simulink library "OutputBlocks_library"  (R2018b)
settings: Solver=VariableStepAuto  StartTime=0.0  StopTime=10.0  RelTol=1e-3
undefined symbols (not defined in the file): aircraft
libraries: unit_conversions_lib x8, flight_parameters_lib x3, vlm_wing_lib x3, axes_transformation_lib x2, sensors_lib x1, flight_dynamics_models x1
settings Model: ModifiedByFormat=dcava  Creator=cava_da  LastModifiedBy=dcava
settings DataIOCC: ReturnWorkspaceOutputs=on

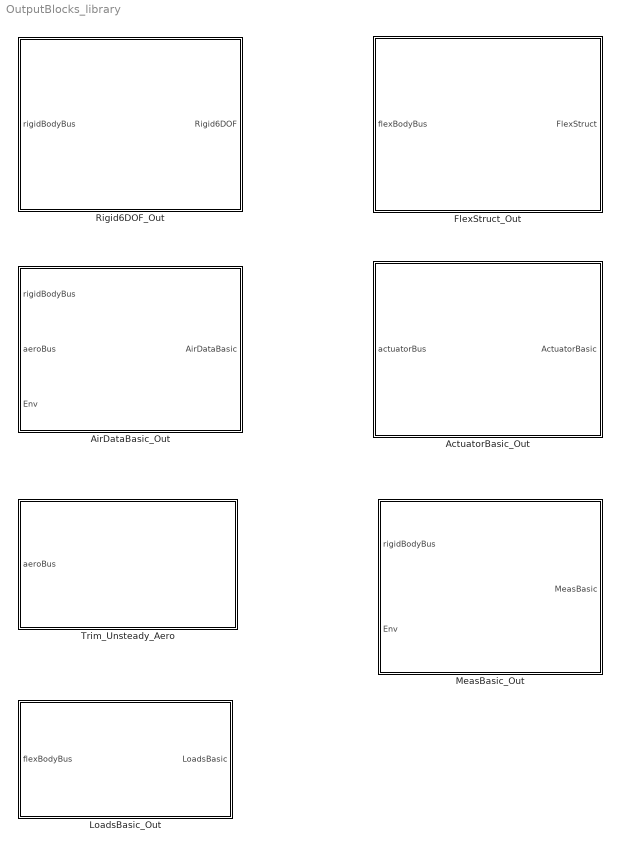
== system OutputBlocks_library ==
  ActuatorBasic_Out : Subsystem  mask{n_ail_pairs=aircraft.wing_main.params.num_flaps/2}
      mask prompts: n_ail_pairs "Number of aileron pairs:"
  AirDataBasic_Out : Subsystem  mask(AirDataBasic_Out){}
      mask DialogControl DescGroupVar Prompt: Air Data Basic
  FlexStruct_Out : Subsystem  mask(FlexStruct_Out){structure_order=size(aircraft.eom_flexible.structure_red.K,2)-6.}
      mask prompts: structure_order "Structural model order"
      mask DialogControl DescGroupVar Prompt: FlexStruct_Out
  LoadsBasic_Out : Subsystem  mask(LoadsBasic_Out){struct_order=size(aircraft.eom_flexible.structure_red.K,2)-6., phi_loads=aircraft.outputs.loads.phi}
      mask prompts: struct_order "Structural model order"; phi_loads "Load transformation matrix (phi)"
  MeasBasic_Out : Subsystem  mask(Rigid6DOF_Out){}
  Rigid6DOF_Out : Subsystem  mask(Rigid6DOF_Out){}
  Trim_Unsteady_Aero : Subsystem  mask{aircraft=aircraft}
      mask prompts: aircraft "Aircraft parameters struct, see aircraftSe2aCreate"
      mask DialogControl DescGroupVar Prompt: Trim Unsteady Aero

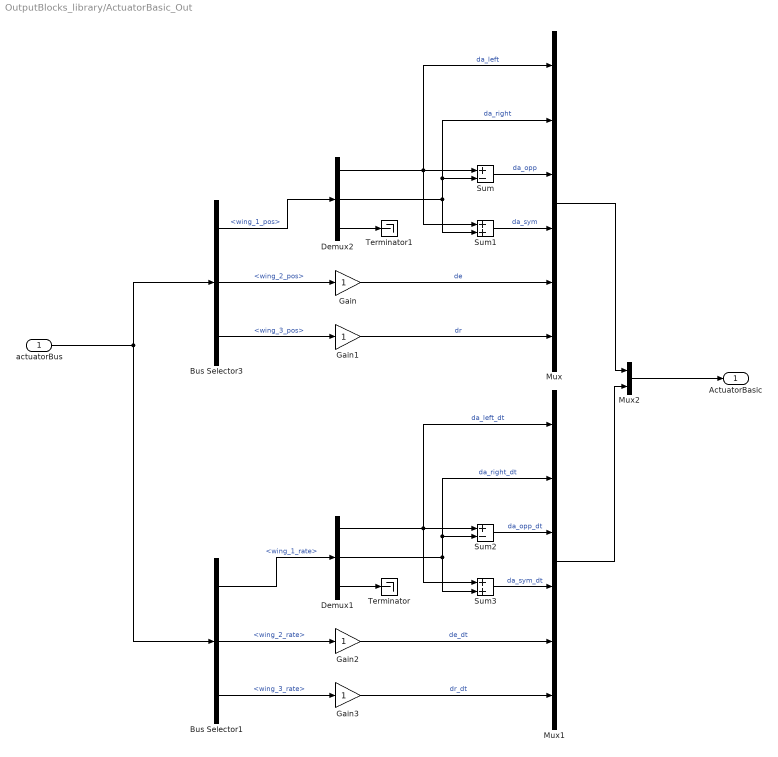
== system OutputBlocks_library/ActuatorBasic_Out ==
  actuatorBus : Inport
  Bus Selector1 : BusSelector  OutputSignals=wing_1_rate,wing_2_rate,wing_3_rate
  Bus Selector3 : BusSelector  OutputSignals=wing_1_pos,wing_2_pos,wing_3_pos
  Demux1 : Demux  Outputs=[n_ail_pairs n_ail_pairs -1]
  Demux2 : Demux  Outputs=[n_ail_pairs n_ail_pairs -1]
  Gain{,1..3} (4 alike) : Gain
  Mux : Mux  Inputs=6
  Mux1 : Mux  Inputs=6
  Mux2 : Mux  Inputs=2
  Sum : Sum  Inputs=+-
  Sum1 : Sum
  Sum2 : Sum  Inputs=+-
  Sum3 : Sum
  Terminator : Terminator
  Terminator1 : Terminator
  ActuatorBasic : Outport  VectorParamsAs1DForOutWhenUnconnected=off
  wires:
  Demux2/3 -> Terminator1/1
  Bus Selector3/1 -> Demux2/1  "<wing_1_pos>"
  Demux1/3 -> Terminator/1
  Bus Selector3/2 -> Gain/1  "<wing_2_pos>"
  Mux/1 -> Mux2/1
  actuatorBus/1 -> Bus Selector1/1, Bus Selector3/1
  Demux2/1 -> Sum1/1, Sum/1, Mux/1  "da_left"
  Demux2/2 -> Sum1/2, Sum/2, Mux/2  "da_right"
  Sum/1 -> Mux/3  "da_opp"
  Sum1/1 -> Mux/4  "da_sym"
  Gain/1 -> Mux/5  "de"
  Bus Selector3/3 -> Gain1/1  "<wing_3_pos>"
  Gain1/1 -> Mux/6  "dr"
  Gain2/1 -> Mux1/5  "de_dt"
  Mux1/1 -> Mux2/2
  Sum3/1 -> Mux1/4  "da_sym_dt"
  Sum2/1 -> Mux1/3  "da_opp_dt"
  Demux1/1 -> Sum2/1, Mux1/1, Sum3/1  "da_left_dt"
  Demux1/2 -> Sum2/2, Mux1/2, Sum3/2  "da_right_dt"
  Gain3/1 -> Mux1/6  "dr_dt"
  Bus Selector1/3 -> Gain3/1  "<wing_3_rate>"
  Bus Selector1/2 -> Gain2/1  "<wing_2_rate>"
  Bus Selector1/1 -> Demux1/1  "<wing_1_rate>"
  Mux2/1 -> ActuatorBasic/1

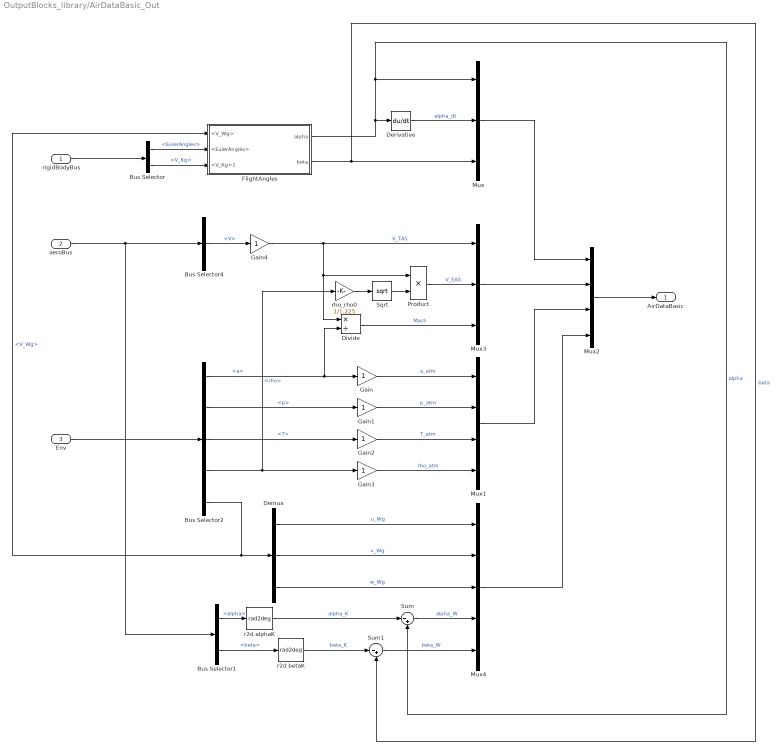
== system OutputBlocks_library/AirDataBasic_Out ==
  rigidBodyBus : Inport
  aeroBus : Inport  Port=2
  Env : Inport  Port=3
  Bus Selector : BusSelector  OutputSignals=EulerAngles,V_Kg
  Bus Selector1 : BusSelector  OutputSignals=main.body.alpha,main.body.beta
  Bus Selector2 : BusSelector  OutputSignals=envir.atmosphere.a,envir.atmosphere.p,envir.atmosphere.T,envir.atmosphere.rho,envir.wind.V_Wg
  Bus Selector4 : BusSelector  OutputSignals=main.body.V
  Demux : Demux  Outputs=3
  Derivative : Derivative  CoefficientInTFapproximation=0.001
  Divide : Product  Inputs=*/
  FlightAngles : Subsystem
  Gain{,1..4} (5 alike) : Gain
  Mux : Mux  Inputs=3
  Mux1 : Mux
  Mux2 : Mux
  Mux3 : Mux  Inputs=3
  Mux4 : Mux  Inputs=5
  Product : Product
  Sqrt : Sqrt  SaturateOnIntegerOverflow=on
  Sum : Sum  Inputs=|-+
  Sum1 : Sum  Inputs=|-+
  r2d alphaK : unit_conversions_lib/rad2deg
      settings: SourceProductName=LADAC
  r2d betaK : unit_conversions_lib/rad2deg
      settings: SourceProductName=LADAC
  rho_rho0 : Gain  Gain=1/1.225
  AirDataBasic : Outport  VectorParamsAs1DForOutWhenUnconnected=off
  wires:
  r2d betaK/1 -> Sum1/1  "beta_K"
  r2d alphaK/1 -> Sum/1  "alpha_K"
  Sum/1 -> Mux4/4  "alpha_W"
  Sum1/1 -> Mux4/5  "beta_W"
  rigidBodyBus/1 -> Bus Selector/1
  Bus Selector1/2 -> r2d betaK/1  "<beta>"
  Bus Selector1/1 -> r2d alphaK/1  "<alpha>"
  Bus Selector/2 -> FlightAngles/3(<V_Kg>1)  "<V_Kg>"
  FlightAngles/1(alpha) -> Derivative/1, Sum/2, Mux/1  "alpha"
  Bus Selector/1 -> FlightAngles/2(<EulerAngles>)  "<EulerAngles>"
  Gain4/1 -> Divide/1, Product/1, Mux3/1  "V_TAS"
  Mux4/1 -> Mux2/4
  Gain3/1 -> Mux1/4  "rho_atm"
  Gain2/1 -> Mux1/3  "T_atm"
  Gain1/1 -> Mux1/2  "p_atm"
  Gain/1 -> Mux1/1  "a_atm"
  Mux3/1 -> Mux2/2
  Mux2/1 -> AirDataBasic/1
  Mux/1 -> Mux2/1
  Mux1/1 -> Mux2/3
  Demux/3 -> Mux4/3  "w_Wg"
  Demux/2 -> Mux4/2  "v_Wg"
  Demux/1 -> Mux4/1  "u_Wg"
  Divide/1 -> Mux3/3  "Mach"
  Bus Selector2/5 -> Demux/1, FlightAngles/1(<V_Wg>)  "<V_Wg>"
  Bus Selector2/4 -> rho_rho0/1, Gain3/1  "<rho>"
  Bus Selector2/3 -> Gain2/1  "<T>"
  Bus Selector2/2 -> Gain1/1  "<p>"
  Bus Selector2/1 -> Gain/1, Divide/2  "<a>"
  Env/1 -> Bus Selector2/1
  FlightAngles/2(beta) -> Sum1/2, Mux/3  "beta"
  Bus Selector4/1 -> Gain4/1  "<V>"
  Derivative/1 -> Mux/2  "alpha_dt"
  aeroBus/1 -> Bus Selector1/1, Bus Selector4/1
  rho_rho0/1 -> Sqrt/1
  Sqrt/1 -> Product/2
  Product/1 -> Mux3/2  "V_EAS"

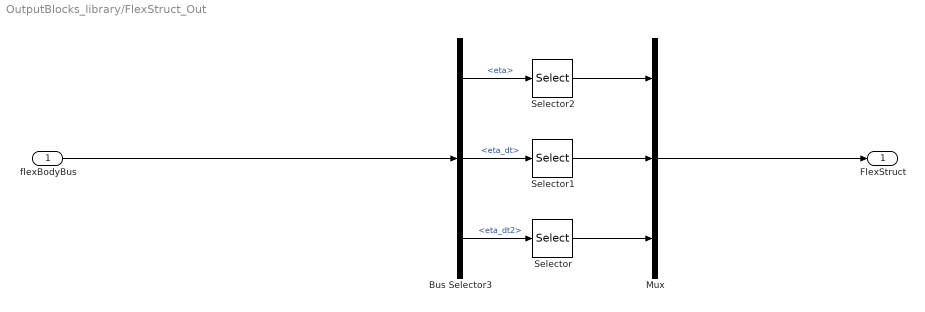
== system OutputBlocks_library/FlexStruct_Out ==
  flexBodyBus : Inport
  Bus Selector3 : BusSelector  OutputSignals=eta,eta_dt,eta_dt2
  Mux : Mux  Inputs=3
  Selector : Selector  InputPortWidth=structure_order+6  IndexOptions=Index vector (dialog)  Indices=7:(structure_order+6)  OutputSizes=1
  Selector1 : Selector  InputPortWidth=structure_order+6  IndexOptions=Index vector (dialog)  Indices=7:(structure_order+6)  OutputSizes=1
  Selector2 : Selector  InputPortWidth=structure_order+6  IndexOptions=Index vector (dialog)  Indices=7:(structure_order+6)  OutputSizes=1
  FlexStruct : Outport  VectorParamsAs1DForOutWhenUnconnected=off
  wires:
  Bus Selector3/3 -> Selector/1  "<eta_dt2>"
  Bus Selector3/1 -> Selector2/1  "<eta>"
  Bus Selector3/2 -> Selector1/1  "<eta_dt>"
  Mux/1 -> FlexStruct/1
  flexBodyBus/1 -> Bus Selector3/1
  Selector/1 -> Mux/3
  Selector1/1 -> Mux/2
  Selector2/1 -> Mux/1

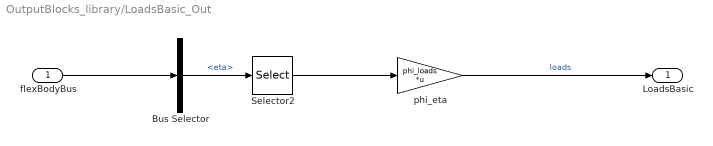
== system OutputBlocks_library/LoadsBasic_Out ==
  flexBodyBus : Inport
  Bus Selector : BusSelector  OutputSignals=eta
  Selector2 : Selector  InputPortWidth=struct_order+6  IndexOptions=Index vector (dialog)  Indices=7:(struct_order+6)  OutputSizes=1
  phi_eta : Gain  Gain=phi_loads  Multiplication=Matrix(K*u)
  LoadsBasic : Outport  VectorParamsAs1DForOutWhenUnconnected=off
  wires:
  phi_eta/1 -> LoadsBasic/1  "loads"
  Bus Selector/1 -> Selector2/1  "<eta>"
  flexBodyBus/1 -> Bus Selector/1
  Selector2/1 -> phi_eta/1

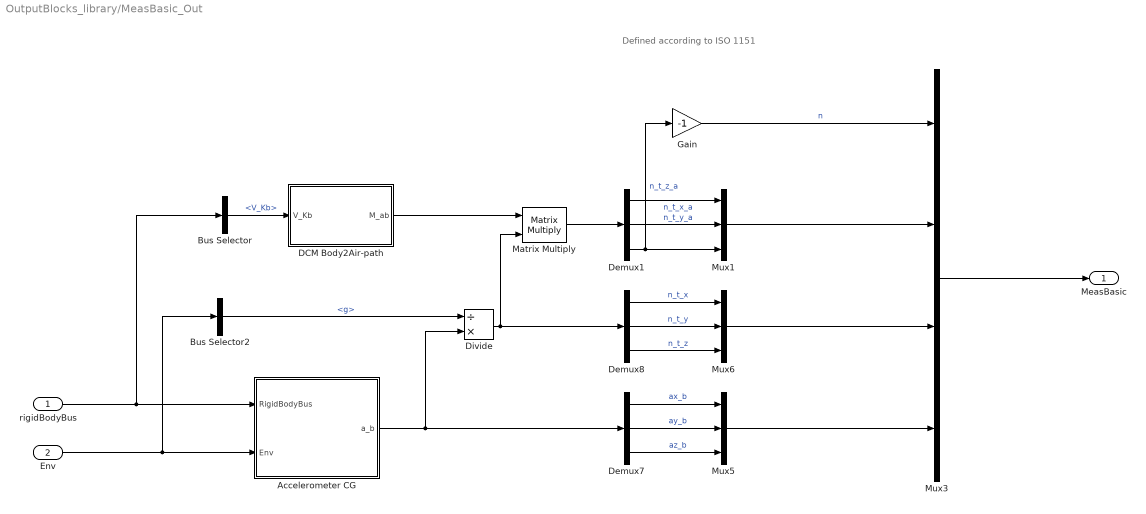
== system OutputBlocks_library/MeasBasic_Out ==
  note: Defined according to ISO 1151
  rigidBodyBus : Inport
  Env : Inport  Port=2
  Accelerometer CG : Subsystem
  Bus Selector : BusSelector  OutputSignals=V_Kb
  Bus Selector2 : BusSelector  OutputSignals=envir.g
  DCM Body2Air-path : Subsystem
  Demux1 : Demux  Outputs=3
  Demux7 : Demux  Outputs=3
  Demux8 : Demux  Outputs=3
  Divide : Product  Inputs=/*
  Gain : Gain  Gain=-1
  Matrix Multiply : Product  Multiplication=Matrix(*)
  Mux1 : Mux  Inputs=3
  Mux3 : Mux
  Mux5 : Mux  Inputs=3
  Mux6 : Mux  Inputs=3
  MeasBasic : Outport  VectorParamsAs1DForOutWhenUnconnected=off
  wires:
  Demux8/1 -> Mux6/1  "n_t_x"
  Divide/1 -> Matrix Multiply/2, Demux8/1
  Demux8/2 -> Mux6/2  "n_t_y"
  Demux8/3 -> Mux6/3  "n_t_z"
  Demux7/3 -> Mux5/3  "az_b"
  Demux7/2 -> Mux5/2  "ay_b"
  Demux7/1 -> Mux5/1  "ax_b"
  Mux3/1 -> MeasBasic/1
  DCM Body2Air-path/1(M_ab) -> Matrix Multiply/1
  Matrix Multiply/1 -> Demux1/1
  Demux1/3 -> Mux1/3, Gain/1  "n_t_z_a"
  Demux1/2 -> Mux1/2  "n_t_y_a"
  Demux1/1 -> Mux1/1  "n_t_x_a"
  Gain/1 -> Mux3/1  "n"
  Accelerometer CG/1(a_b) -> Divide/2, Demux7/1
  rigidBodyBus/1 -> Bus Selector/1, Accelerometer CG/1(RigidBodyBus)
  Env/1 -> Bus Selector2/1, Accelerometer CG/2(Env)
  Bus Selector/1 -> DCM Body2Air-path/1(V_Kb)  "<V_Kb>"
  Bus Selector2/1 -> Divide/1  "<g>"
  Mux1/1 -> Mux3/2
  Mux6/1 -> Mux3/3
  Mux5/1 -> Mux3/4

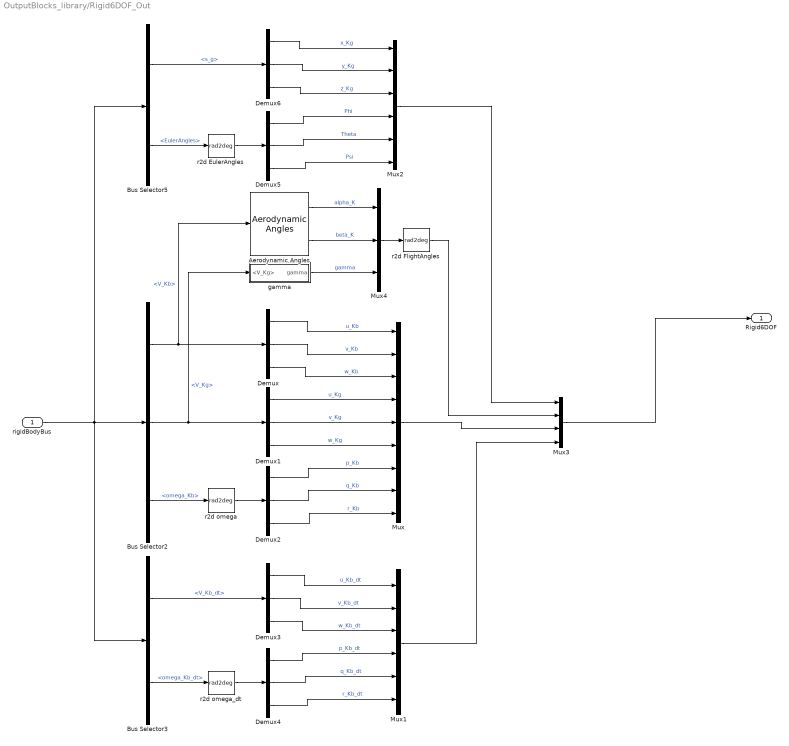
== system OutputBlocks_library/Rigid6DOF_Out ==
  rigidBodyBus : Inport
  Aerodynamic Angles : flight_parameters_lib/Aerodynamic Angles  SystemSampleTime=-1  Latency=0  AutoFrameSizeCalculation=off
      settings: SourceProductName=LADAC
  Bus Selector2 : BusSelector  OutputSignals=V_Kb,V_Kg,omega_Kb
  Bus Selector3 : BusSelector  OutputSignals=V_Kb_dt,omega_Kb_dt
  Bus Selector5 : BusSelector  OutputSignals=s_g,EulerAngles
  Demux{,1..6} (7 alike) : Demux  Outputs=3
  Mux : Mux  Inputs=9
  Mux1 : Mux  Inputs=6
  Mux2 : Mux  Inputs=6
  Mux3 : Mux
  Mux4 : Mux  Inputs=3
  gamma : Subsystem
  r2d EulerAngles : unit_conversions_lib/rad2deg
      settings: SourceProductName=LADAC
  r2d FlightAngles : unit_conversions_lib/rad2deg
      settings: SourceProductName=LADAC
  r2d omega : unit_conversions_lib/rad2deg
      settings: SourceProductName=LADAC
  r2d omega_dt : unit_conversions_lib/rad2deg
      settings: SourceProductName=LADAC
  Rigid6DOF : Outport  VectorParamsAs1DForOutWhenUnconnected=off
  wires:
  Mux4/1 -> r2d FlightAngles/1
  gamma/1(gamma) -> Mux4/3  "gamma"
  Aerodynamic Angles/2 -> Mux4/2  "beta_K"
  Aerodynamic Angles/1 -> Mux4/1  "alpha_K"
  r2d FlightAngles/1 -> Mux3/2
  rigidBodyBus/1 -> Bus Selector3/1, Bus Selector5/1, Bus Selector2/1
  Demux5/1 -> Mux2/4  "Phi"
  Demux3/2 -> Mux1/2  "v_Kb_dt"
  Bus Selector2/2 -> Demux1/1, gamma/1(<V_Kg>)  "<V_Kg>"
  Bus Selector3/1 -> Demux3/1  "<V_Kb_dt>"
  Mux1/1 -> Mux3/4
  Bus Selector3/2 -> r2d omega_dt/1  "<omega_Kb_dt>"
  Demux2/1 -> Mux/7  "p_Kb"
  Demux4/3 -> Mux1/6  "r_Kb_dt"
  Demux6/3 -> Mux2/3  "z_Kg"
  Demux5/3 -> Mux2/6  "Psi"
  Demux4/1 -> Mux1/4  "p_Kb_dt"
  Demux6/1 -> Mux2/1  "x_Kg"
  Mux/1 -> Mux3/3
  Demux1/1 -> Mux/4  "u_Kg"
  Demux2/3 -> Mux/9  "r_Kb"
  Demux1/3 -> Mux/6  "w_Kg"
  Demux/3 -> Mux/3  "w_Kb"
  Bus Selector5/1 -> Demux6/1  "<s_g>"
  Demux1/2 -> Mux/5  "v_Kg"
  Demux/2 -> Mux/2  "v_Kb"
  Demux2/2 -> Mux/8  "q_Kb"
  Bus Selector5/2 -> r2d EulerAngles/1  "<EulerAngles>"
  Demux3/1 -> Mux1/1  "u_Kb_dt"
  Demux/1 -> Mux/1  "u_Kb"
  Bus Selector2/1 -> Demux/1, Aerodynamic Angles/1  "<V_Kb>"
  Mux2/1 -> Mux3/1
  Demux4/2 -> Mux1/5  "q_Kb_dt"
  Demux5/2 -> Mux2/5  "Theta"
  Demux6/2 -> Mux2/2  "y_Kg"
  Bus Selector2/3 -> r2d omega/1  "<omega_Kb>"
  Demux3/3 -> Mux1/3  "w_Kb_dt"
  Mux3/1 -> Rigid6DOF/1
  r2d EulerAngles/1 -> Demux5/1
  r2d omega/1 -> Demux2/1
  r2d omega_dt/1 -> Demux4/1

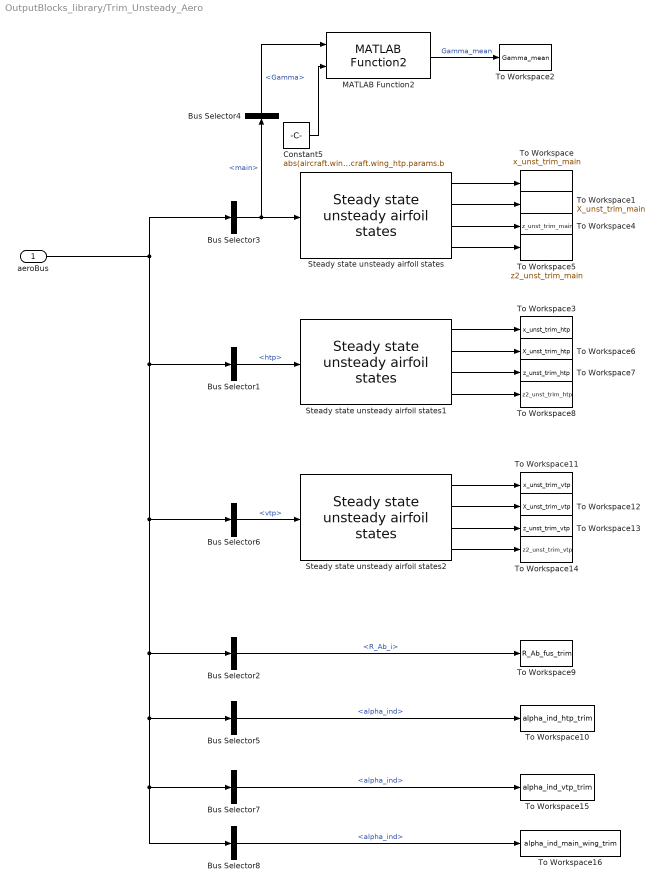
== system OutputBlocks_library/Trim_Unsteady_Aero ==
  aeroBus : Inport
  Bus Selector1 : BusSelector  OutputSignals=htp
  Bus Selector2 : BusSelector  OutputSignals=fuselage.aero.R_Ab_i
  Bus Selector3 : BusSelector  OutputSignals=main
  Bus Selector4 : BusSelector  OutputSignals=aero.circulation.Gamma
  Bus Selector5 : BusSelector  OutputSignals=htp.aero.circulation.alpha_ind
  Bus Selector6 : BusSelector  OutputSignals=vtp
  Bus Selector7 : BusSelector  OutputSignals=vtp.aero.circulation.alpha_ind
  Bus Selector8 : BusSelector  OutputSignals=main.aero.circulation.alpha_ind
  Constant5 : Constant  Value=abs(aircraft.wing_main.geometry.ctrl_pt.pos(2,:))<aircraft.wing_htp.params.b
  MATLAB Function2 : flight_dynamics_models/Flexible aircraft with steady aerodynamics/Aerodynamics/MATLAB Function2  SystemSampleTime=-1  Latency=0  AutoFrameSizeCalculation=off
      settings: SourceProductName=SE2A library
  Steady state unsteady airfoil states : vlm_wing_lib/Steady state unsteady airfoil states  wing_airfoil=aircraft.wing_main.airfoil  wing_config=aircraft.wing_main.config
      settings: SourceProductName=LADAC
  Steady state unsteady airfoil states1 : vlm_wing_lib/Steady state unsteady airfoil states  wing_airfoil=aircraft.wing_htp.airfoil  wing_config=aircraft.wing_htp.config
      settings: SourceProductName=LADAC
  Steady state unsteady airfoil states2 : vlm_wing_lib/Steady state unsteady airfoil states  wing_airfoil=aircraft.wing_vtp.airfoil  wing_config=aircraft.wing_vtp.config
      settings: SourceProductName=LADAC
  To Workspace : ToWorkspace  VariableName=x_unst_trim_main  SampleTime=-1
      settings: MaxDataPoints=8  Save2DSignal=2-D array (concatenate along first dimension)
  To Workspace1 : ToWorkspace  VariableName=X_unst_trim_main  SampleTime=-1
      settings: MaxDataPoints=3  Save2DSignal=2-D array (concatenate along first dimension)
  To Workspace10 : ToWorkspace  VariableName=alpha_ind_htp_trim  SampleTime=-1
      settings: MaxDataPoints=1  Save2DSignal=2-D array (concatenate along first dimension)
  To Workspace11 : ToWorkspace  VariableName=x_unst_trim_vtp  SampleTime=-1
      settings: MaxDataPoints=8  Save2DSignal=2-D array (concatenate along first dimension)
  To Workspace12 : ToWorkspace  VariableName=X_unst_trim_vtp  SampleTime=-1
      settings: MaxDataPoints=3  Save2DSignal=2-D array (concatenate along first dimension)
  To Workspace13 : ToWorkspace  VariableName=z_unst_trim_vtp  SampleTime=-1
      settings: MaxDataPoints=2  Save2DSignal=2-D array (concatenate along first dimension)
  To Workspace14 : ToWorkspace  VariableName=z2_unst_trim_vtp  SampleTime=-1
      settings: MaxDataPoints=1
  To Workspace15 : ToWorkspace  VariableName=alpha_ind_vtp_trim  SampleTime=-1
      settings: MaxDataPoints=1  Save2DSignal=2-D array (concatenate along first dimension)
  To Workspace16 : ToWorkspace  VariableName=alpha_ind_main_wing_trim  SampleTime=-1
      settings: MaxDataPoints=1  Save2DSignal=2-D array (concatenate along first dimension)
  To Workspace2 : ToWorkspace  VariableName=Gamma_mean  SampleTime=-1
      settings: MaxDataPoints=1
  To Workspace3 : ToWorkspace  VariableName=x_unst_trim_htp  SampleTime=-1
      settings: MaxDataPoints=8  Save2DSignal=2-D array (concatenate along first dimension)
  To Workspace4 : ToWorkspace  VariableName=z_unst_trim_main  SampleTime=-1
      settings: MaxDataPoints=2  Save2DSignal=2-D array (concatenate along first dimension)
  To Workspace5 : ToWorkspace  VariableName=z2_unst_trim_main  SampleTime=-1
      settings: MaxDataPoints=1
  To Workspace6 : ToWorkspace  VariableName=X_unst_trim_htp  SampleTime=-1
      settings: MaxDataPoints=3  Save2DSignal=2-D array (concatenate along first dimension)
  To Workspace7 : ToWorkspace  VariableName=z_unst_trim_htp  SampleTime=-1
      settings: MaxDataPoints=2  Save2DSignal=2-D array (concatenate along first dimension)
  To Workspace8 : ToWorkspace  VariableName=z2_unst_trim_htp  SampleTime=-1
      settings: MaxDataPoints=1
  To Workspace9 : ToWorkspace  VariableName=R_Ab_fus_trim  SampleTime=-1
      settings: MaxDataPoints=3  Save2DSignal=2-D array (concatenate along first dimension)
  wires:
  Constant5/1 -> MATLAB Function2/2
  Steady state unsteady airfoil states/3 -> To Workspace4/1
  Steady state unsteady airfoil states/2 -> To Workspace1/1
  Bus Selector3/1 -> Steady state unsteady airfoil states/1, Bus Selector4/1  "<main>"
  Bus Selector4/1 -> MATLAB Function2/1  "<Gamma>"
  Steady state unsteady airfoil states/1 -> To Workspace/1
  MATLAB Function2/1 -> To Workspace2/1  "Gamma_mean"
  Steady state unsteady airfoil states/4 -> To Workspace5/1
  Steady state unsteady airfoil states1/4 -> To Workspace8/1
  Steady state unsteady airfoil states1/1 -> To Workspace3/1
  Steady state unsteady airfoil states1/2 -> To Workspace6/1
  Steady state unsteady airfoil states1/3 -> To Workspace7/1
  Bus Selector1/1 -> Steady state unsteady airfoil states1/1  "<htp>"
  Bus Selector2/1 -> To Workspace9/1  "<R_Ab_i>"
  Bus Selector5/1 -> To Workspace10/1  "<alpha_ind>"
  aeroBus/1 -> Bus Selector6/1, Bus Selector8/1, Bus Selector7/1, Bus Selector5/1, Bus Selector2/1, Bus Selector1/1, Bus Selector3/1
  Bus Selector6/1 -> Steady state unsteady airfoil states2/1  "<vtp>"
  Steady state unsteady airfoil states2/3 -> To Workspace13/1
  Steady state unsteady airfoil states2/2 -> To Workspace12/1
  Steady state unsteady airfoil states2/1 -> To Workspace11/1
  Steady state unsteady airfoil states2/4 -> To Workspace14/1
  Bus Selector7/1 -> To Workspace15/1  "<alpha_ind>"
  Bus Selector8/1 -> To Workspace16/1  "<alpha_ind>"

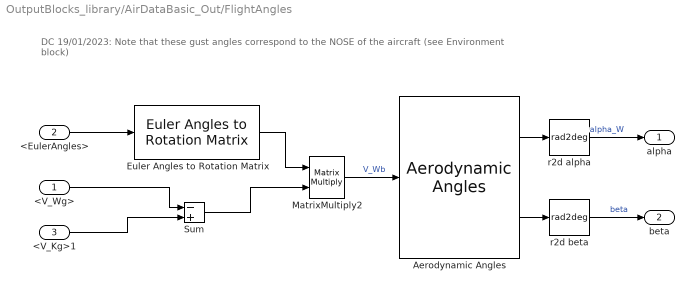
== system OutputBlocks_library/AirDataBasic_Out/FlightAngles ==
  note: DC 19/01/2023: Note that these gust angles correspond to the NOSE of the aircraft (see Environment block)
  <V_Wg> : Inport
  <EulerAngles> : Inport  Port=2
  <V_Kg>1 : Inport  Port=3
  Aerodynamic Angles : flight_parameters_lib/Aerodynamic Angles  SystemSampleTime=-1  Latency=0  AutoFrameSizeCalculation=off
      settings: SourceProductName=LADAC
  Euler Angles to Rotation Matrix : axes_transformation_lib/Euler Angles to Rotation Matrix  SystemSampleTime=-1  Latency=0  AutoFrameSizeCalculation=off
      settings: SourceProductName=LADAC
  MatrixMultiply2 : Product  Multiplication=Matrix(*)
  Sum : Sum  Inputs=-+
  r2d alpha : unit_conversions_lib/rad2deg
      settings: SourceProductName=LADAC
  r2d beta : unit_conversions_lib/rad2deg
      settings: SourceProductName=LADAC
  alpha : Outport  VectorParamsAs1DForOutWhenUnconnected=off
  beta : Outport  Port=2  VectorParamsAs1DForOutWhenUnconnected=off
  wires:
  Sum/1 -> MatrixMultiply2/2
  r2d beta/1 -> beta/1  "beta"
  r2d alpha/1 -> alpha/1  "alpha_W"
  <V_Wg>/1 -> Sum/1
  MatrixMultiply2/1 -> Aerodynamic Angles/1  "V_Wb"
  Aerodynamic Angles/1 -> r2d alpha/1
  Euler Angles to Rotation Matrix/1 -> MatrixMultiply2/1
  <EulerAngles>/1 -> Euler Angles to Rotation Matrix/1
  Aerodynamic Angles/2 -> r2d beta/1
  <V_Kg>1/1 -> Sum/2

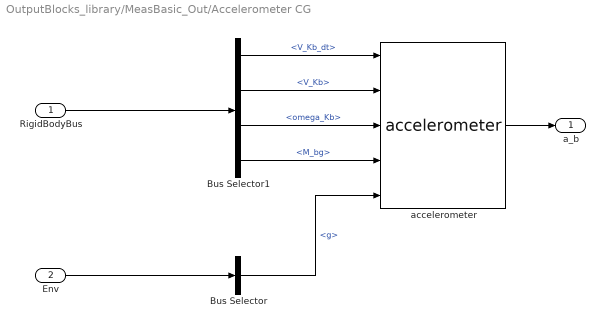
== system OutputBlocks_library/MeasBasic_Out/Accelerometer CG ==
  RigidBodyBus : Inport
  Env : Inport  Port=2
  Bus Selector : BusSelector  OutputSignals=envir.g
  Bus Selector1 : BusSelector  OutputSignals=V_Kb_dt,V_Kb,omega_Kb,M_bg
  accelerometer : sensors_lib/accelerometer  SystemSampleTime=-1  Latency=0  AutoFrameSizeCalculation=off
      settings: SourceProductName=LADAC
  a_b : Outport  VectorParamsAs1DForOutWhenUnconnected=off
  wires:
  Bus Selector/1 -> accelerometer/5  "<g>"
  accelerometer/1 -> a_b/1
  Bus Selector1/3 -> accelerometer/3  "<omega_Kb>"
  Bus Selector1/1 -> accelerometer/1  "<V_Kb_dt>"
  Bus Selector1/4 -> accelerometer/4  "<M_bg>"
  RigidBodyBus/1 -> Bus Selector1/1
  Env/1 -> Bus Selector/1
  Bus Selector1/2 -> accelerometer/2  "<V_Kb>"

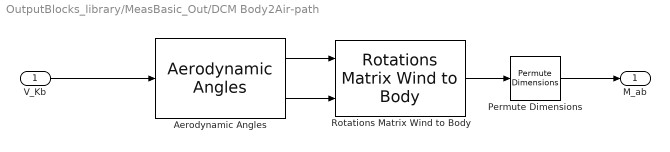
== system OutputBlocks_library/MeasBasic_Out/DCM Body2Air-path ==
  V_Kb : Inport
  Aerodynamic Angles : flight_parameters_lib/Aerodynamic Angles  SystemSampleTime=-1  Latency=0  AutoFrameSizeCalculation=off
      settings: SourceProductName=LADAC
  Permute Dimensions : PermuteDimensions
  Rotations Matrix Wind to Body : axes_transformation_lib/Rotations Matrix Wind to Body  SystemSampleTime=-1  Latency=0  AutoFrameSizeCalculation=off
      settings: SourceProductName=LADAC
  M_ab : Outport  VectorParamsAs1DForOutWhenUnconnected=off
  wires:
  Aerodynamic Angles/2 -> Rotations Matrix Wind to Body/2
  Rotations Matrix Wind to Body/1 -> Permute Dimensions/1
  Permute Dimensions/1 -> M_ab/1
  Aerodynamic Angles/1 -> Rotations Matrix Wind to Body/1
  V_Kb/1 -> Aerodynamic Angles/1

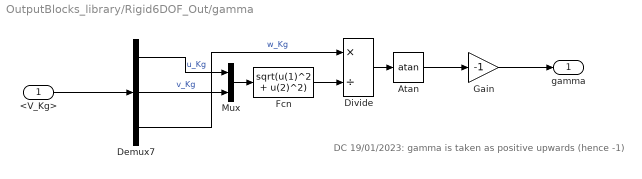
== system OutputBlocks_library/Rigid6DOF_Out/gamma ==
  note: DC 19/01/2023: gamma is taken as positive upwards (hence -1)
  <V_Kg> : Inport
  Atan : Trigonometry  Operator=atan
  Demux7 : Demux  Outputs=3
  Divide : Product  Inputs=*/
  Fcn : Fcn  Expr=sqrt(u(1)^2 + u(2)^2)
  Gain : Gain  Gain=-1
  Mux : Mux  Inputs=2
  gamma : Outport  VectorParamsAs1DForOutWhenUnconnected=off
  wires:
  Gain/1 -> gamma/1
  Fcn/1 -> Divide/2
  Mux/1 -> Fcn/1
  Demux7/2 -> Mux/2  "v_Kg"
  Atan/1 -> Gain/1
  Demux7/1 -> Mux/1  "u_Kg"
  Demux7/3 -> Divide/1  "w_Kg"
  Divide/1 -> Atan/1
  <V_Kg>/1 -> Demux7/1
